simulink model "ps04_ex3_LinearModel"  (R2021b)
settings: Solver=ode4  StartTime=0.0  StopTime=100  FixedStep=0.001  RelTol=1e-3
values from neighbouring files (symbols this model uses):
  K_mpc = M*((Theta'*Gamma'*Q*Gamma*Theta+R)\(Theta'*Gamma'*Q))    [ps04_run_ex1.m]
undefined symbols (not defined in the file or in its folder): linearizationPt, Psi, sysC, Upsilon
settings Model: Creator=rihutter  LastModifiedBy=rafis
settings SolverCC: AlgebraicLoopSolver=TrustRegion
settings DataIOCC: ReturnWorkspaceOutputs=off
settings DebuggingCC: SFMachineParentedDataDiag=warning  ArithmeticOperatorsInVariantConditions=warning
settings SFSimCC: SimUseLocalCustomCode=off  CustomCodeUndefinedFunction=UseInterfaceOnly
settings RTWCC: RTWUseLocalCustomCode=off
settings CodeAppCC: StateflowObjectComments=on

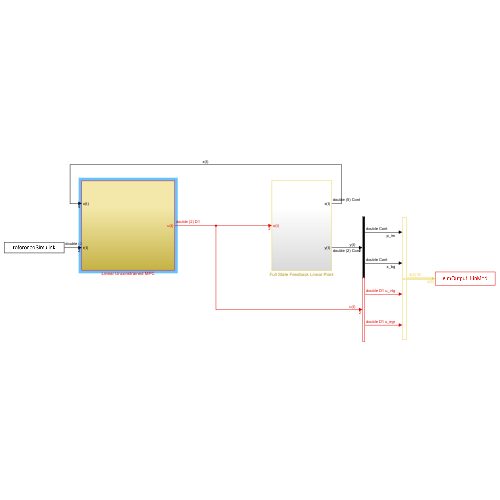
[thumbnail: Simulink's stored preview of the top-level diagram]
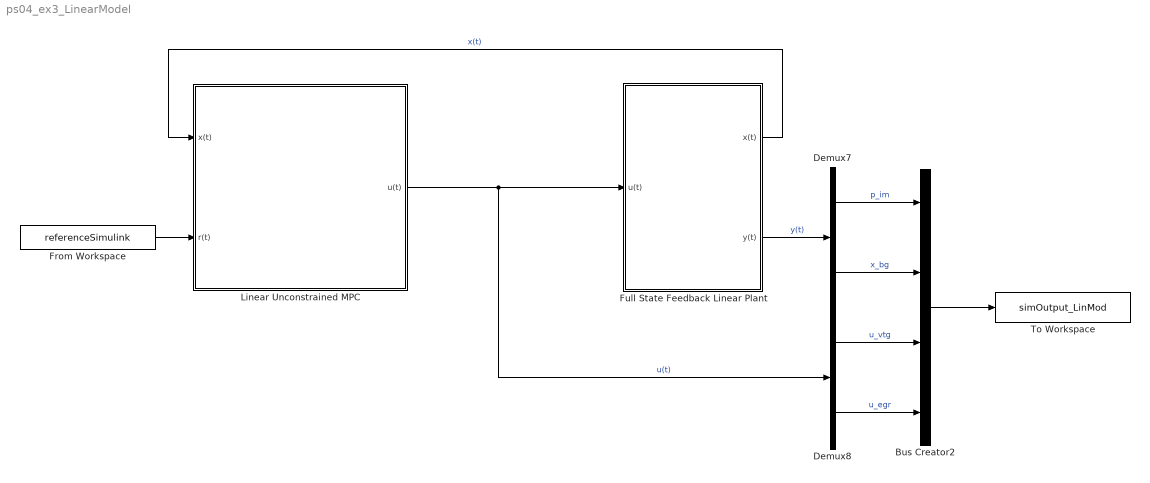
== system ps04_ex3_LinearModel ==
  Bus Creator2 : BusCreator  Inputs=4
  Demux7 : Demux  Outputs=2
  Demux8 : Demux  Outputs=2
  From Workspace : FromWorkspace  VariableName=referenceSimulink  Interpolate=off  OutputAfterFinalValue=Holding final value
  Full State Feedback Linear Plant : Subsystem
  Linear Unconstrained MPC : Subsystem
  To Workspace : ToWorkspace  VariableName=simOutput_LinMod  SaveFormat=Timeseries  SampleTime=-1
  wires:
  From Workspace/1 -> Linear Unconstrained MPC/2(r(t))
  Linear Unconstrained MPC/1(u(t)) -> Demux8/1, Full State Feedback Linear Plant/1(u(t))  "u(t)"
  Full State Feedback Linear Plant/2(y(t)) -> Demux7/1  "y(t)"
  Bus Creator2/1 -> To Workspace/1
  Demux7/1 -> Bus Creator2/1  "p_im"
  Demux7/2 -> Bus Creator2/2  "x_bg"
  Demux8/1 -> Bus Creator2/3  "u_vtg"
  Demux8/2 -> Bus Creator2/4  "u_egr"
  Full State Feedback Linear Plant/1(x(t)) -> Linear Unconstrained MPC/1(x(t))  "x(t)"

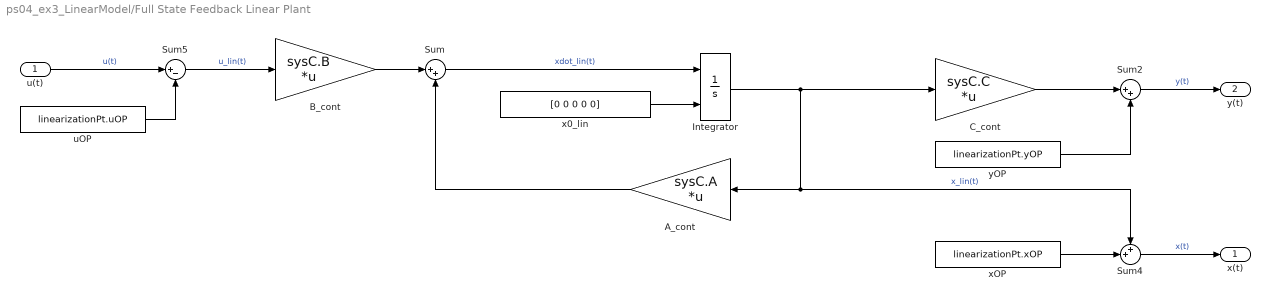
== system ps04_ex3_LinearModel/Full State Feedback Linear Plant ==
  u(t) : Inport
  A_cont : Gain  Gain=sysC.A  Multiplication=Matrix(K*u)
  B_cont : Gain  Gain=sysC.B  Multiplication=Matrix(K*u)
  C_cont : Gain  Gain=sysC.C  Multiplication=Matrix(K*u)
  Integrator : Integrator  InitialConditionSource=external
  Sum : Sum  Inputs=|++
  Sum2 : Sum  Inputs=|++
  Sum4 : Sum  Inputs=++|
  Sum5 : Sum  Inputs=|+-
  uOP : Constant  Value=linearizationPt.uOP
  x0_lin : Constant  Value=[0 0 0 0 0]
  xOP : Constant  Value=linearizationPt.xOP
  yOP : Constant  Value=linearizationPt.yOP
  x(t) : Outport  VectorParamsAs1DForOutWhenUnconnected=off
  y(t) : Outport  Port=2  VectorParamsAs1DForOutWhenUnconnected=off
  wires:
  Sum2/1 -> y(t)/1  "y(t)"
  C_cont/1 -> Sum2/1
  yOP/1 -> Sum2/2
  Sum5/1 -> B_cont/1  "u_lin(t)"
  xOP/1 -> Sum4/2
  Sum4/1 -> x(t)/1  "x(t)"
  u(t)/1 -> Sum5/1  "u(t)"
  uOP/1 -> Sum5/2
  Integrator/1 -> Sum4/1, A_cont/1, C_cont/1  "x_lin(t)"
  x0_lin/1 -> Integrator/2
  B_cont/1 -> Sum/1
  Sum/1 -> Integrator/1  "xdot_lin(t)"
  A_cont/1 -> Sum/2

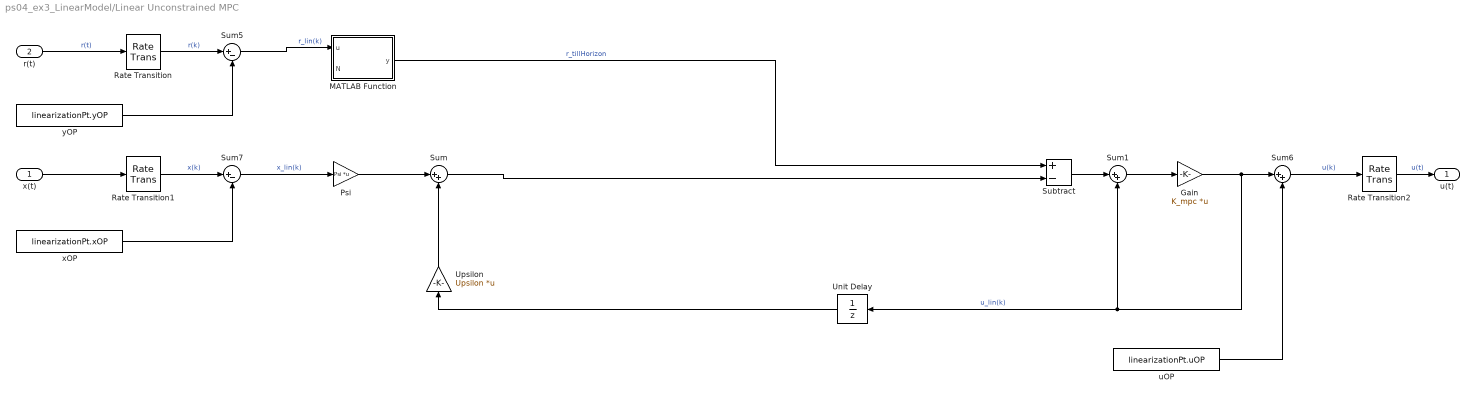
== system ps04_ex3_LinearModel/Linear Unconstrained MPC ==
  x(t) : Inport
  r(t) : Inport  Port=2
  Gain : Gain  Gain=K_mpc  Multiplication=Matrix(K*u)
  MATLAB Function : MATLAB Function  TreatAsAtomicUnit=on
  Psi : Gain  Gain=Psi  Multiplication=Matrix(K*u)
  Rate Transition : RateTransition  OutPortSampleTime=0.05
  Rate Transition1 : RateTransition  OutPortSampleTime=0.05
  Rate Transition2 : RateTransition  InitialCondition=linearizationPt.uOP
  Subtract : Sum  Inputs=+-
  Sum : Sum  Inputs=|++
  Sum1 : Sum  Inputs=|++
  Sum5 : Sum  Inputs=|+-
  Sum6 : Sum  Inputs=|++
  Sum7 : Sum  Inputs=|+-
  Unit Delay : UnitDelay  SampleTime=-1  HasFrameUpgradeWarning=on
  Upsilon : Gain  Gain=Upsilon  Multiplication=Matrix(K*u)
  uOP : Constant  Value=linearizationPt.uOP
  xOP : Constant  Value=linearizationPt.xOP
  yOP : Constant  Value=linearizationPt.yOP
  u(t) : Outport  VectorParamsAs1DForOutWhenUnconnected=off
  wires:
  yOP/1 -> Sum5/2
  Sum6/1 -> Rate Transition2/1  "u(k)"
  uOP/1 -> Sum6/2
  xOP/1 -> Sum7/2
  x(t)/1 -> Rate Transition1/1
  r(t)/1 -> Rate Transition/1  "r(t)"
  Rate Transition/1 -> Sum5/1  "r(k)"
  Rate Transition1/1 -> Sum7/1  "x(k)"
  Rate Transition2/1 -> u(t)/1  "u(t)"
  Sum5/1 -> MATLAB Function/1(u)  "r_lin(k)"
  Sum7/1 -> Psi/1  "x_lin(k)"
  Gain/1 -> Sum1/2, Unit Delay/1, Sum6/1  "u_lin(k)"
  MATLAB Function/1(y) -> Subtract/1  "r_tillHorizon"
  Upsilon/1 -> Sum/2
  Psi/1 -> Sum/1
  Sum/1 -> Subtract/2
  Subtract/1 -> Sum1/1
  Unit Delay/1 -> Upsilon/1
  Sum1/1 -> Gain/1

== matlab function ps04_ex3_LinearModel/Linear Unconstrained MPC/MATLAB Function ==
  data: u input; y output; N input
function y = fcn(u,N)

y = repmat(u,50,1);
